simulink model "nonlinearPlnt_ul_th"  (R2018a)
settings: Solver=FixedStepAuto  StartTime=0.0  StopTime=simulationDuration_s  FixedStep=simulationTimeStep_s  RelTol=1e-3
libraries: nonlinearPlnt_ul x1
settings Model: Creator=mcobb  LastModifiedBy=mcobb

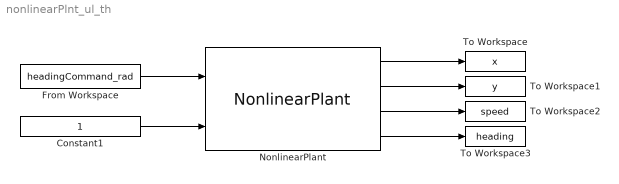
== system nonlinearPlnt_ul_th ==
  Constant1 : Constant
  From Workspace : FromWorkspace  VariableName=headingCommand_rad  SampleTime=0
  NonlinearPlant : nonlinearPlnt_ul/NonlinearPlant
  To Workspace : ToWorkspace  VariableName=x  SaveFormat=Timeseries  SampleTime=-1
  To Workspace1 : ToWorkspace  VariableName=y  SaveFormat=Timeseries  SampleTime=-1
  To Workspace2 : ToWorkspace  VariableName=speed  SaveFormat=Timeseries  SampleTime=-1
  To Workspace3 : ToWorkspace  VariableName=heading  SaveFormat=Timeseries  SampleTime=-1
  wires:
  From Workspace/1 -> NonlinearPlant/1
  Constant1/1 -> NonlinearPlant/2
  NonlinearPlant/1 -> To Workspace/1
  NonlinearPlant/2 -> To Workspace1/1
  NonlinearPlant/3 -> To Workspace2/1
  NonlinearPlant/4 -> To Workspace3/1
